simulink model "x2goldcode"  (R2023b)
settings: Solver=FixedStepDiscrete  StartTime=0.0  StopTime=10.0  RelTol=1e-3
libraries: commseqgen3 x3
settings Model: Creator=The MathWorks, Inc.  LastModifiedBy=Abhi Singh
settings SolverCC: AlgebraicLoopSolver=TrustRegion
settings DebuggingCC: UnconnectedInputMsg=warning  UnconnectedOutputMsg=warning  UnconnectedLineMsg=warning
settings ModelReferenceCC: EnableRefExpFcnMdlSchedulingChecks=on
settings RTWCC: DLArmComputeVersion=19.05

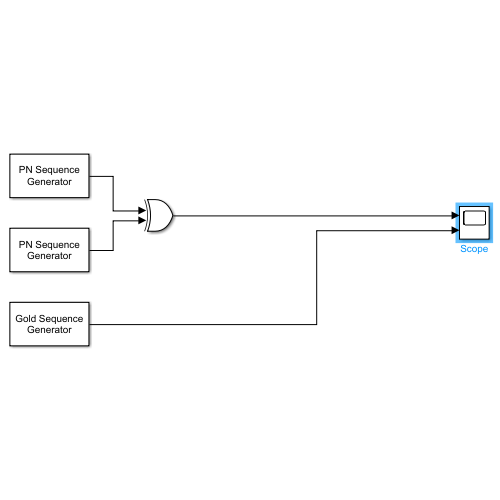
[thumbnail: Simulink's stored preview of the top-level diagram]
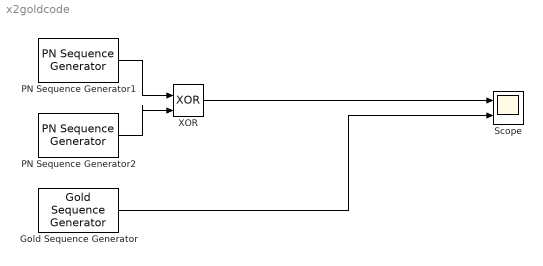
== system x2goldcode ==
  Gold Sequence Generator : commseqgen3/Gold Sequence Generator  genPoly1=[5 2 0]  iniState1=[0 0 0 0 1]  genPoly2=[5 4 3 2 0]  iniState2=[0 0 0 0 1]  index=0  shift=0  outVarSiz=off  maxOutSizeMode=Dialog parameter  maxOutSize=[10 1]  Ts=1  sampPerFrame=1  reset=off  outDataType=double
  PN Sequence Generator1 : commseqgen3/PN Sequence Generator  poly=[5 2 0]  ini_sta=[0 0 0 0 1]  outBitMaskSource=Dialog parameter  shift=0  outVarSiz=off  maxOutSizeMode=Dialog parameter  maxOutSize=[10 1]  Ts=1  sampPerFrame=1  reset=off  bitPackedOutputs=off  outDataType=double  numPackedBits=8  bitPackDataSigned=off  bitPackedOutDType=double
  PN Sequence Generator2 : commseqgen3/PN Sequence Generator  poly=[5 4 3 2 0]  ini_sta=[0 0 0 0 1]  outBitMaskSource=Dialog parameter  shift=0  outVarSiz=off  maxOutSizeMode=Dialog parameter  maxOutSize=[10 1]  Ts=1  sampPerFrame=1  reset=off  bitPackedOutputs=off  outDataType=double  numPackedBits=8  bitPackDataSigned=off  bitPackedOutDType=double
  Scope : Scope  NumInputPorts=2
  XOR : Logic  Operator=XOR  IconShape=distinctive  AllPortsSameDT=off  OutDataTypeStr=float('double')
  wires:
  PN Sequence Generator1/1 -> XOR/1
  PN Sequence Generator2/1 -> XOR/2
  XOR/1 -> Scope/1
  Gold Sequence Generator/1 -> Scope/2
